simulink model "cps_cameras_v2"  (R2012b)
settings: Solver=FixedStepDiscrete  StartTime=0.0  StopTime=8.5  RelTol=20e-5
model workspace (MAT data in the model file):
  ini_nozzle_vpos = 0.3
  ini_B_block_vpos = 0.01
  ini_G_block_vpos = 0.11
  block_height = 0.3
values from neighbouring files (symbols this model uses):
  useStereopsis = 1    [cps_workspace_variables_v2.mat]
libraries: cps_lib_v2 x3, vrlib x3, simulink x1
settings Model: Creator=pmosterm  LastModifiedBy=pmosterm
settings SolverCC: ZcThreshold=2e-5  MaxConsecutiveZCs=20  EnableConcurrentExecution=on  ConcurrentTasks=on  ZeroCrossAlgorithm=Adaptive  SolverResetMethod=Robust
settings DataIOCC: SignalLogging=off
settings OptimizationCC: InlineParams=on
settings DebuggingCC: ReadBeforeWriteMsg=DisableAll  WriteAfterWriteMsg=DisableAll  WriteAfterReadMsg=DisableAll  AlgebraicLoopMsg=error  UnderspecifiedInitializationDetection=Simplified  FcnCallInpInsideContextMsg=EnableAllAsWarning  ModelReferenceExtraNoncontSigs=warning
settings GRTTargetCC: CombineOutputUpdateFcns=off  GRTInterface=on
settings ConfigurationSet: Description=SimMechanics 2G

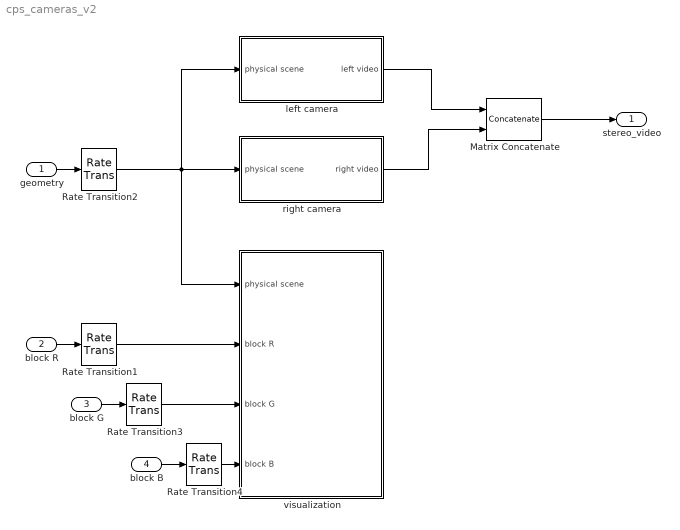
== system cps_cameras_v2 ==
  geometry : Inport  OutDataTypeStr=Bus: slBusGeometry  SampleTime=0.005
  block R : Inport  Port=2  OutDataTypeStr=Bus: slBusBlockOps  SampleTime=0.05  BusOutputAsStruct=on
  block G : Inport  Port=3  OutDataTypeStr=Bus: slBusBlockOps  SampleTime=0.05  BusOutputAsStruct=on
  block B : Inport  Port=4  OutDataTypeStr=Bus: slBusBlockOps  SampleTime=0.05  BusOutputAsStruct=on
  Matrix Concatenate : Concatenate  Mode=Multidimensional array  ConcatenateDimension=3
  Rate Transition{1..4} (4 alike) : RateTransition  Deterministic=off  OutPortSampleTime=0.1
  left camera : Subsystem  Variant=on
  right camera : Subsystem  Variant=on
  visualization : Subsystem
  stereo_video : Outport
  wires:
  geometry/1 -> Rate Transition2/1
  left camera/1(left video) -> Matrix Concatenate/1
  right camera/1(right video) -> Matrix Concatenate/2
  Matrix Concatenate/1 -> stereo_video/1
  block G/1 -> Rate Transition3/1
  block R/1 -> Rate Transition1/1
  block B/1 -> Rate Transition4/1
  Rate Transition2/1 -> right camera/1(physical scene), left camera/1(physical scene), visualization/1(physical scene)
  Rate Transition1/1 -> visualization/2(block R)
  Rate Transition3/1 -> visualization/3(block G)
  Rate Transition4/1 -> visualization/4(block B)

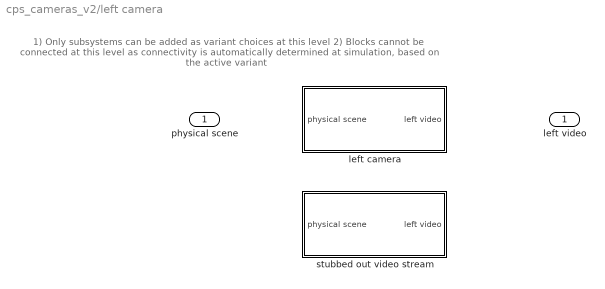
== system cps_cameras_v2/left camera ==
  note: 1) Only subsystems can be added as variant choices at this level
      | 2) Blocks cannot be connected at this level as connectivity is
      | automatically determined at simulation, based on the active variant
  physical scene : Inport
  left camera : Subsystem  VariantObject=useStereopsisVariant
  stubbed out video stream : Subsystem  VariantObject=noStereopsisVariant
  left video : Outport

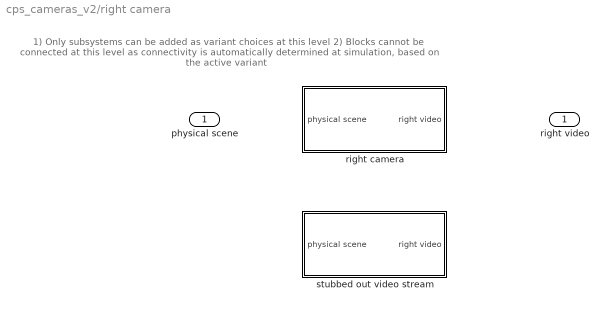
== system cps_cameras_v2/right camera ==
  note: 1) Only subsystems can be added as variant choices at this level
      | 2) Blocks cannot be connected at this level as connectivity is
      | automatically determined at simulation, based on the active variant
  physical scene : Inport
  right camera : Subsystem  VariantObject=useStereopsisVariant
  stubbed out video stream : Subsystem  VariantObject=noStereopsisVariant
  right video : Outport

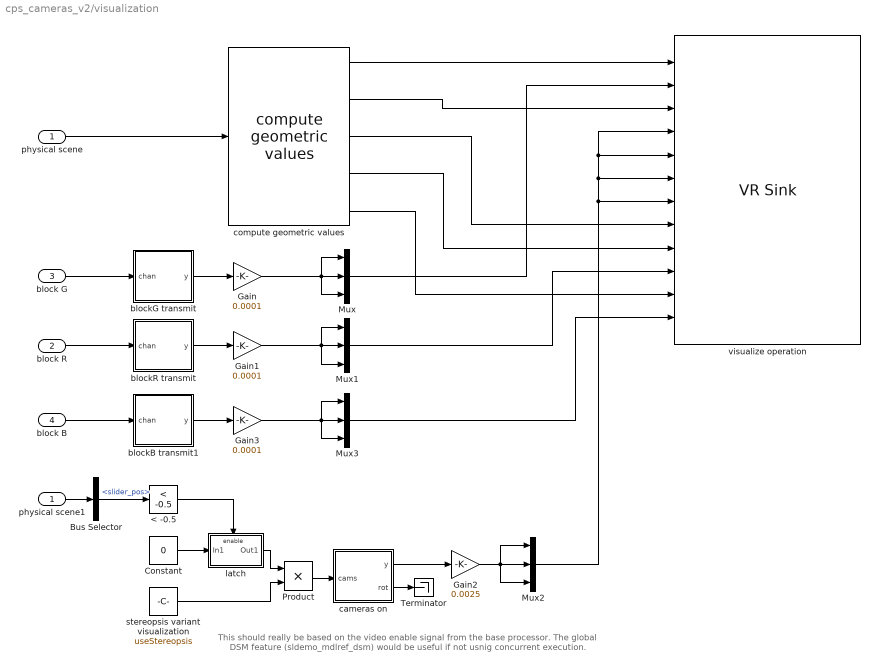
== system cps_cameras_v2/visualization ==
  note: This should really be based on the video enable
      | signal from the base processor.
      | The global DSM feature (sldemo_mdlref_dsm) would
      | be useful if not usnig concurrent execution.
  physical scene : Inport
  block R : Inport  Port=2  OutDataTypeStr=Bus: slBusBlockOps  BusOutputAsStruct=on
  block G : Inport  Port=3  OutDataTypeStr=Bus: slBusBlockOps  BusOutputAsStruct=on
  block B : Inport  Port=4  OutDataTypeStr=Bus: slBusBlockOps  BusOutputAsStruct=on
  < -0.5 : simulink/Logic and Bit Operations/Compare To Constant  relop=<  const=-0.5  OutDataTypeStr=boolean
  Bus Selector : BusSelector  OutputSignals=slider_pos
  Constant : Constant  Value=0  OutDataTypeStr=Inherit: Inherit via back propagation
  Gain : Gain  Gain=0.0001
  Gain1 : Gain  Gain=0.0001
  Gain2 : Gain  Gain=0.0025
  Gain3 : Gain  Gain=0.0001
  Mux{,1..3} (4 alike) : Mux  Inputs=3
  Product : Product  OutDataTypeStr=uint8  RndMeth=Zero
  Terminator : Terminator
  blockB transmit1 : Stateflow chart  TreatAsAtomicUnit=on
  blockG transmit : Stateflow chart  TreatAsAtomicUnit=on
  blockR transmit : Stateflow chart  TreatAsAtomicUnit=on
  cameras on : Stateflow chart  TreatAsAtomicUnit=on
  compute geometric values : cps_lib_v2/compute geometric values
  latch : Subsystem  TreatAsAtomicUnit=on
  physical scene1 : InportShadow
  stereopsis variant visualization : Constant  Value=useStereopsis  OutDataTypeStr=Inherit: Inherit via back propagation
  visualize operation : vrlib/VR Sink  InstantiateOnLoad=on  SampleTime=0.1  ViewEnable=on  RemoteChange=off  RemoteView=off  FieldsWritten=red_block2x3dim.translation.3.1.1.double#blockG_waves.scale.3.1.1.double#slider.translation.3.1.1.double#left_cone_half_one.scale.3.1.1.double#left_cone_half_two.scale.3.1.1.double#right_cone_half_one.scale.3.1.1.double#right_cone_half_two.scale.3.1.1.double#LOWER.translation.3.1.1.double#purple_block2x3dim.translation.3.1.1.double#blockR_waves.scale.3.1.1.double#blue_block2x3dim.translation.3.1.1.double#blockB_waves.scale.3.1.1.double  WorldFileName=cps_world_v2x.wrl  AutoView=on  VideoDimensions=[]  AllowVariableSize=off  FigureProperties="{'Position', 'Name', 'Viewpoint', 'CameraBound', 'CameraDirection', 'CameraPosition', 'CameraUpVector', 'ZoomFactor', 'Antialiasing', 'Headlight', 'Lighting', 'NavPanel', 'StatusBar', 'ToolBar', 'Textures', 'Transparency', 'Triad', 'Wireframe', 'NavZones', 'NavMode', 'NavSpeed', 'CaptureFileFormat', 'CaptureFileName', 'Record2DCompressMethod', 'Record2DCompressQuality', 'Record2D', 'Record2DFileName', 'Record2DFPS'; [1.9000000000000000e+01   5.6800000000000000e+02   5.7600000000000000e+02   3.8000000000000000e+02], '', 'front', 'on', [0.0000000000000000e+00   0.0000000000000000e+00  -1.0000000000000000e+00], [0.0000000000000000e+00   0.0000000000000000e+00   0.0000000000000000e+00], [0.0000000000000000e+00   1.0000000000000000e+00   0.0000000000000000e+00], [1.0000000000000000e+00], 'on', 'on', 'on', 'halfbar', 'on', 'on', 'on', 'on', 'none', 'off', 'off', 'walk', 'normal', 'tif', '%f_anim_%n.tif', 'auto', [7.5000000000000000e+01], 'off', '%f_anim_%n.avi', [1.5000000000000000e+01]}"
  wires:
  physical scene/1 -> compute geometric values/1
  blockG transmit/1(y) -> Gain/1
  Gain/1 -> Mux/3, Mux/1, Mux/2
  blockR transmit/1(y) -> Gain1/1
  Gain1/1 -> Mux1/3, Mux1/1, Mux1/2
  block G/1 -> blockG transmit/1(chan)
  physical scene1/1 -> Bus Selector/1
  Bus Selector/1 -> < -0.5/1  "<slider_pos>"
  Constant/1 -> latch/1(In1)
  < -0.5/1 -> latch/Enable
  cameras on/1(y) -> Gain2/1
  Gain2/1 -> Mux2/1, Mux2/2, Mux2/3
  cameras on/2(rot) -> Terminator/1
  Product/1 -> cameras on/1(cams)
  latch/1(Out1) -> Product/1
  stereopsis variant visualization/1 -> Product/2
  compute geometric values/1 -> visualize operation/1
  Mux/1 -> visualize operation/2
  compute geometric values/2 -> visualize operation/3
  Mux2/1 -> visualize operation/4, visualize operation/5, visualize operation/6, visualize operation/7
  compute geometric values/3 -> visualize operation/8
  compute geometric values/4 -> visualize operation/9
  Mux1/1 -> visualize operation/10
  compute geometric values/5 -> visualize operation/11
  blockB transmit1/1(y) -> Gain3/1
  Gain3/1 -> Mux3/2, Mux3/1, Mux3/3
  block B/1 -> blockB transmit1/1(chan)
  Mux3/1 -> visualize operation/12
  block R/1 -> blockR transmit/1(chan)

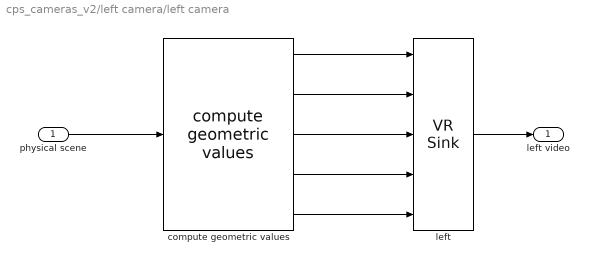
== system cps_cameras_v2/left camera/left camera ==
  physical scene : Inport
  compute geometric values : cps_lib_v2/compute geometric values
  left : vrlib/VR Sink  InstantiateOnLoad=on  SampleTime=0.1  ViewEnable=on  RemoteChange=off  RemoteView=off  FieldsWritten=red_block2x3dim.translation.3.1.1.double#slider.translation.3.1.1.double#LOWER.translation.3.1.1.double#purple_block2x3dim.translation.3.1.1.double#blue_block2x3dim.translation.3.1.1.double  WorldFileName=cps_world_v2.wrl  AutoView=off  VideoDimensions=[400 240]  AllowVariableSize=off  FigureProperties="{'Position', 'Name', 'Viewpoint', 'CameraBound', 'CameraDirection', 'CameraPosition', 'CameraUpVector', 'ZoomFactor', 'Antialiasing', 'Headlight', 'Lighting', 'NavPanel', 'StatusBar', 'ToolBar', 'Textures', 'Transparency', 'Triad', 'Wireframe', 'NavZones', 'NavMode', 'NavSpeed', 'CaptureFileFormat', 'CaptureFileName', 'Record2DCompressMethod', 'Record2DCompressQuality', 'Record2D', 'Record2DFileName', 'Record2DFPS'; [8.9500000000000000e+02   6.0000000000000000e+01   2.4000000000000000e+02   4.0000000000000000e+02], '', 'left', 'on', [0.0000000000000000e+00   0.0000000000000000e+00  -1.0000000000000000e+00], [0.0000000000000000e+00   0.0000000000000000e+00   0.0000000000000000e+00], [0.0000000000000000e+00   1.0000000000000000e+00   0.0000000000000000e+00], [1.0000000000000000e+00], 'on', 'on', 'on', 'none', 'off', 'off', 'on', 'on', 'none', 'off', 'off', 'walk', 'normal', 'tif', '%f_anim_%n.tif', 'auto', [7.5000000000000000e+01], 'off', '***video***', [1.5000000000000000e+01]}"
  left video : Outport
  wires:
  left/1 -> left video/1
  physical scene/1 -> compute geometric values/1
  compute geometric values/3 -> left/3
  compute geometric values/4 -> left/4
  compute geometric values/2 -> left/2
  compute geometric values/5 -> left/5
  compute geometric values/1 -> left/1

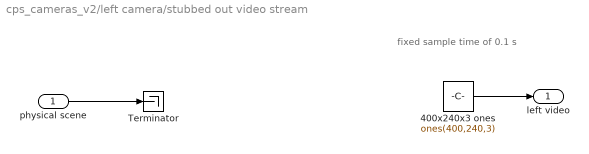
== system cps_cameras_v2/left camera/stubbed out video stream ==
  note: fixed sample time
      | of 0.1 s
  physical scene : Inport
  400x240x3 ones : Constant  Value=ones(400,240,3)  VectorParams1D=off  OutDataTypeStr=uint8  SampleTime=0.1
  Terminator : Terminator
  left video : Outport
  wires:
  400x240x3 ones/1 -> left video/1
  physical scene/1 -> Terminator/1

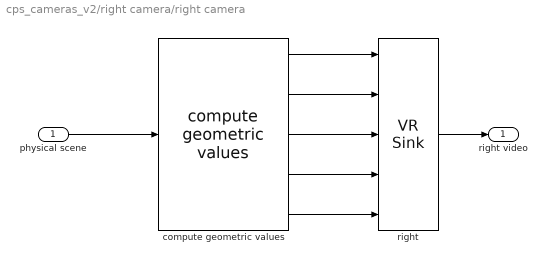
== system cps_cameras_v2/right camera/right camera ==
  physical scene : Inport
  compute geometric values : cps_lib_v2/compute geometric values
  right : vrlib/VR Sink  InstantiateOnLoad=on  SampleTime=0.1  ViewEnable=on  RemoteChange=off  RemoteView=off  FieldsWritten=red_block2x3dim.translation.3.1.1.double#slider.translation.3.1.1.double#LOWER.translation.3.1.1.double#purple_block2x3dim.translation.3.1.1.double#blue_block2x3dim.translation.3.1.1.double  WorldFileName=cps_world_v2.wrl  AutoView=off  VideoDimensions=[400 240]  AllowVariableSize=off  FigureProperties="{'Position', 'Name', 'Viewpoint', 'CameraBound', 'CameraDirection', 'CameraPosition', 'CameraUpVector', 'ZoomFactor', 'Antialiasing', 'Headlight', 'Lighting', 'NavPanel', 'StatusBar', 'ToolBar', 'Textures', 'Transparency', 'Triad', 'Wireframe', 'NavZones', 'NavMode', 'NavSpeed', 'CaptureFileFormat', 'CaptureFileName', 'Record2DCompressMethod', 'Record2DCompressQuality', 'Record2D', 'Record2DFileName', 'Record2DFPS'; [1.1400000000000000e+03   6.0000000000000000e+01   2.4000000000000000e+02   4.0000000000000000e+02], '', 'right', 'on', [0.0000000000000000e+00   0.0000000000000000e+00  -1.0000000000000000e+00], [0.0000000000000000e+00   0.0000000000000000e+00   0.0000000000000000e+00], [0.0000000000000000e+00   1.0000000000000000e+00   0.0000000000000000e+00], [1.0000000000000000e+00], 'on', 'on', 'on', 'none', 'off', 'off', 'on', 'on', 'none', 'off', 'off', 'walk', 'normal', 'tif', '%f_anim_%n.tif', 'auto', [7.5000000000000000e+01], 'off', '***video***', [1.5000000000000000e+01]}"
  right video : Outport
  wires:
  physical scene/1 -> compute geometric values/1
  right/1 -> right video/1
  compute geometric values/3 -> right/3
  compute geometric values/2 -> right/2
  compute geometric values/4 -> right/4
  compute geometric values/5 -> right/5
  compute geometric values/1 -> right/1

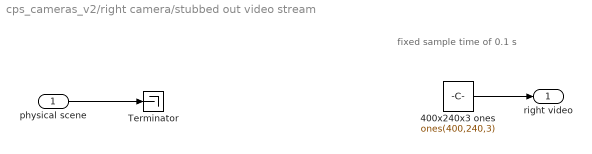
== system cps_cameras_v2/right camera/stubbed out video stream ==
  note: fixed sample time
      | of 0.1 s
  physical scene : Inport
  400x240x3 ones : Constant  Value=ones(400,240,3)  VectorParams1D=off  OutDataTypeStr=uint8  SampleTime=0.1
  Terminator : Terminator
  right video : Outport
  wires:
  400x240x3 ones/1 -> right video/1
  physical scene/1 -> Terminator/1

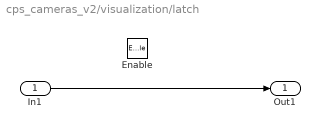
== system cps_cameras_v2/visualization/latch ==
  In1 : Inport
  Enable : EnablePort
  Out1 : Outport  InitialOutput=1
  wires:
  In1/1 -> Out1/1

== stateflow chart cps_cameras_v2/visualization/blockR transmit ==
  state A
    en: y = 1;
  state B
    en: y = 2;
  state C
    en: y = 3;
  state D
    en: y = 4;
  state E
    en: y = 5;
  (default) -> A : /y=1;
  (junction 23) -> A
  (junction 22) -> (junction 23)
  A -> B : [chan.moveBlock.move]
  B -> C : [y == 2]
  C -> D : [y == 3]
  D -> E : [y == 4]
  E -> (junction 22) : [y == 5]
  data: y output double; chan input Bus: slBusBlockOps

== stateflow chart cps_cameras_v2/visualization/cameras on ==
  state A
    en:
    y = 0;
    rot = 0;
  state B
    en:
    y = 1;
    rot = 0.31;
  state C
    en:
    y = 2;
    rot = 0.62;
  state D
    en:
    y = 3;
    rot = 0.93;
  state E
    en:
    y = 2;
    rot = 1.24;
  (default) -> A : /y=0;
  (junction 23) -> A
  (junction 30) -> (junction 23) [order 1] : [cams ~= 1]
  A -> B : [cams == 1]
  (junction 30) -> B [order 2] : [cams == 1]
  (junction 22) -> (junction 30)
  B -> C : [y == 1]
  C -> D : [y == 2]
  D -> E : [y == 3]
  E -> (junction 22) : [y == 2]
  data: y output double; cams input; rot output double

== stateflow chart cps_cameras_v2/visualization/blockB transmit1 ==
  state A
    en: y = 1;
  state B
    en: y = 2;
  state C
    en: y = 3;
  state D
    en: y = 4;
  state E
    en: y = 5;
  (default) -> A : /y=1;
  (junction 23) -> A
  (junction 22) -> (junction 23)
  A -> B : [chan.moveBlock.move]
  B -> C : [y == 2]
  C -> D : [y == 3]
  D -> E : [y == 4]
  E -> (junction 22) : [y == 5]
  data: y output double; chan input Bus: slBusBlockOps

== stateflow chart cps_cameras_v2/visualization/blockG transmit ==
  state A
    en: y = 1;
  state B
    en: y = 2;
  state C
    en: y = 3;
  state D
    en: y = 4;
  state E
    en: y = 5;
  (default) -> A : /y=1;
  (junction 23) -> A
  (junction 22) -> (junction 23)
  A -> B : [chan.moveBlock.move]
  B -> C : [y == 2]
  C -> D : [y == 3]
  D -> E : [y == 4]
  E -> (junction 22) : [y == 5]
  data: y output double; chan input Bus: slBusBlockOps
